simulink model "Galvo_sys_cc_neu_norefs_v32"  (R2013a)
settings: Solver=ode23  StartTime=0.0  StopTime=5e-3  MaxStep=1e-5  RelTol=1e-4  AbsTol=1e-6
PreLoadFcn:
  | paramCtrl=evalin('base','paramCtrl;');
  | 
  | I_LIM=str2num(paramCtrl.I_LIM);
  | Kbc=str2num(paramCtrl.Kbc);
InitFcn:
  | %I_LIM=str2num(paramCtrl.I_LIM);
  | %Kbc=str2num(paramCtrl.Kbc);
StartFcn:
  | %I_LIM=str2num(paramCtrl.I_LIM);
  | %Kbc=str2num(paramCtrl.Kbc);
values from neighbouring files (symbols this model uses):
  Lc = 170e-6    (= 0.00017)    [Galvo_process_analyze.m]
  Rc = 1.5    [Galvo_process_analyze.m]
undefined symbols (not defined in the file or in its folder): JR, KBM, KFR, KMT, KTB, Rsh
libraries: simulink x3
settings Model: BufferReuse=off  Creator=mainster  LastModifiedBy=mainster
settings SolverCC: MaxConsecutiveMinStep=2
settings OptimizationCC: BlockReduction=off  OptimizeBlockIOStorage=off  BufferReuse=off  ExpressionFolding=off  LocalBlockOutputs=off
settings ModelReferenceCC: ModelReferenceNumInstancesAllowed=Single

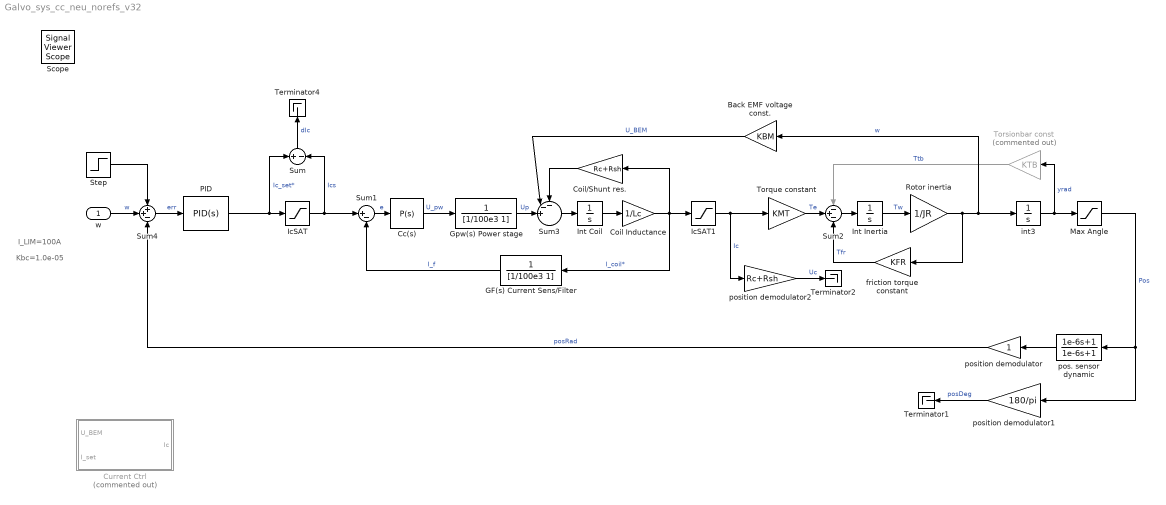
== system Galvo_sys_cc_neu_norefs_v32 ==
  note: I_LIM=100A
  note: Kbc=1.0e-05
  w : Inport
  Back EMF voltage const. : Gain  Gain=KBM
  Cc(s) : simulink/Continuous/PID Controller  Controller=P  TimeDomain=Continuous-time  SampleTime=1  IntegratorMethod=Forward Euler  FilterMethod=Forward Euler  Form=Ideal  P=5.91984122843419  I=14540.01765706  D=0  N=100  InitialConditionSource=internal  InitialConditionForIntegrator=0  InitialConditionForFilter=0  ExternalReset=none  LimitOutput=off  UpperSaturationLimit=inf  LowerSaturationLimit=-inf  LinearizeAsGain=on  AntiWindupMode=none  Kb=1  TrackingMode=off  Kt=1  PParamMin=[]  PParamMax=[]  IParamMin=[]  IParamMax=[]  DParamMin=[]  DParamMax=[]  NParamMin=[]  NParamMax=[]  KbParamMin=[]  KbParamMax=[]  KtParamMin=[]  KtParamMax=[]  POutMin=[]  POutMax=[]  IOutMin=[]  IOutMax=[]  DOutMin=[]  DOutMax=[]  NOutMin=[]  NOutMax=[]  KbOutMin=[]  KbOutMax=[]  KtOutMin=[]  KtOutMax=[]  IntegratorOutMin=[]  IntegratorOutMax=[]  FilterOutMin=[]  FilterOutMax=[]  SumOutMin=[]  SumOutMax=[]  SumI1OutMin=[]  SumI1OutMax=[]  SumI2OutMin=[]  SumI2OutMax=[]  SumI3OutMin=[]  SumI3OutMax=[]  SumDOutMin=[]  SumDOutMax=[]  SaturationOutMin=[]  SaturationOutMax=[]  IntegratorContinuousStateAttributes=''  IntegratorStateMustResolveToSignalObject=off  IntegratorRTWStateStorageClass=Auto  FilterContinuousStateAttributes=''  FilterStateMustResolveToSignalObject=off  FilterRTWStateStorageClass=Auto
  Coil Inductance : Gain  Gain=1/Lc
  Coil/Shunt res. : Gain  Gain=Rc+Rsh
  Current Ctrl : Subsystem  Commented=on
  GF(s) Current Sens/Filter : TransferFcn  Denominator=[1/100e3 1]
  Gpw(s) Power stage : TransferFcn  Denominator=[1/100e3 1]
  IcSAT : Saturate  UpperLimit=I_LIM  LowerLimit=-I_LIM
  IcSAT1 : Saturate  UpperLimit=I_LIM  LowerLimit=-I_LIM
  Int Coil : Integrator
  Int Inertia : Integrator
  Max Angle : Saturate  UpperLimit=20*pi/180  LowerLimit=-20*pi/180
      settings: AttributesFormatString=Max=%<UpperLimit>\nMin=%<LowerLimit>
  PID : simulink/Continuous/PID Controller  Controller=PID  TimeDomain=Continuous-time  SampleTime=1  IntegratorMethod=Forward Euler  FilterMethod=Forward Euler  Form=Ideal  P=5.80637204199794  I=20.9623797027831  D=0.0037150147392085  N=9551.68244277248  InitialConditionSource=internal  InitialConditionForIntegrator=0  InitialConditionForFilter=0  ExternalReset=none  IgnoreLimit=on  LimitOutput=off  UpperSaturationLimit=I_LIM*1e3  LowerSaturationLimit=-I_LIM*1e3  LinearizeAsGain=off  AntiWindupMode=back-calculation  Kb=Kbc  TrackingMode=off  Kt=0  PParamMin=[]  PParamMax=[]  IParamMin=[]  IParamMax=[]  DParamMin=[]  DParamMax=[]  NParamMin=[]  NParamMax=[]  KbParamMin=[]  KbParamMax=[]  KtParamMin=[]  KtParamMax=[]  POutMin=[]  POutMax=[]  IOutMin=[]  IOutMax=[]  DOutMin=[]  DOutMax=[]  NOutMin=[]  NOutMax=[]  KbOutMin=[]  KbOutMax=[]  KtOutMin=[]  KtOutMax=[]  IntegratorOutMin=[]  IntegratorOutMax=[]  FilterOutMin=[]  FilterOutMax=[]  SumOutMin=[]  SumOutMax=[]  SumI1OutMin=[]  SumI1OutMax=[]  SumI2OutMin=[]  SumI2OutMax=[]  SumI3OutMin=[]  SumI3OutMax=[]  SumDOutMin=[]  SumDOutMax=[]  SaturationOutMin=[]  SaturationOutMax=[]  IntegratorContinuousStateAttributes=''  IntegratorStateMustResolveToSignalObject=off  IntegratorRTWStateStorageClass=Auto  FilterContinuousStateAttributes=''  FilterStateMustResolveToSignalObject=off  FilterRTWStateStorageClass=Auto
      settings: AttributesFormatString=AWM=%<AntiWindupMode>\nD=%<D>\nI=%<I>\nN=%<N>\nP=%<P>\nLimit=+-%<UpperSaturationLimit>
  Rotor inertia : Gain  Gain=1/JR
  Step : Step  Time=1e-3  After=1*pi/180  SampleTime=0  ZeroCross=off
      settings: AttributesFormatString=Ampl.: %<After>
  Sum : Sum  Inputs=+-
  Sum1 : Sum  Inputs=|+-
  Sum2 : Sum  Inputs=-+-
  Sum3 : Sum  Inputs=--+||
  Sum4 : Sum  Inputs=++-
  Terminator1 : Terminator
  Terminator2 : Terminator
  Terminator4 : Terminator
  Torque constant : Gain  Gain=KMT
  Torsionbar const : Gain  Commented=on  Gain=KTB
  friction torque constant : Gain  Gain=KFR
  int3 : Integrator
  pos. sensor dynamic : TransferFcn  Numerator=[1e-6 1]  Denominator=[1e-6 1]
  position demodulator : Gain
  position demodulator1 : Gain  Gain=180/pi
  position demodulator2 : Gain  Gain=Rc+Rsh
  Scope : SignalViewerScope  IOType=viewer  NumInputPorts=5  RefreshTime=0.035000
      settings: ShowLegends=on  TimeRange=0.005  YMin=-10~-10~-1~0~-5  YMax=40~50~1~0.2~15
  wires:
  Sum4/1 -> PID/1  "err"
  Step/1 -> Sum4/1
  w/1 -> Sum4/2  "w"
  pos. sensor dynamic/1 -> position demodulator/1
  position demodulator/1 -> Sum4/3  "posRad"
  Max Angle/1 -> position demodulator1/1, pos. sensor dynamic/1  "Pos"
  PID/1 -> Sum/1, IcSAT/1  "Ic_set*"
  Coil Inductance/1 -> IcSAT1/1, Coil/Shunt res./1, GF(s) Current Sens/Filter/1  "I_coil*"
  position demodulator1/1 -> Terminator1/1  "posDeg"
  position demodulator2/1 -> Terminator2/1  "Uc"
  Sum/1 -> Terminator4/1  "dIc"
  IcSAT/1 -> Sum1/1, Sum/2  "Ics"
  Sum1/1 -> Cc(s)/1  "e"
  Coil/Shunt res./1 -> Sum3/1
  Sum3/1 -> Int Coil/1
  Int Coil/1 -> Coil Inductance/1
  Cc(s)/1 -> Gpw(s) Power stage/1  "U_pw"
  Gpw(s) Power stage/1 -> Sum3/3  "Up"
  GF(s) Current Sens/Filter/1 -> Sum1/2  "I_f"
  int3/1 -> Max Angle/1, Torsionbar const/1  "yrad"
  Torque constant/1 -> Sum2/2  "Te"
  Torsionbar const/1 -> Sum2/1  "Ttb"
  Int Inertia/1 -> Rotor inertia/1  "Tw"
  Sum2/1 -> Int Inertia/1
  Rotor inertia/1 -> int3/1, Back EMF voltage const./1, friction torque constant/1  "w"
  friction torque constant/1 -> Sum2/3  "Tfr"
  IcSAT1/1 -> Torque constant/1, position demodulator2/1  "Ic"
  Back EMF voltage const./1 -> Sum3/2  "U_BEM"

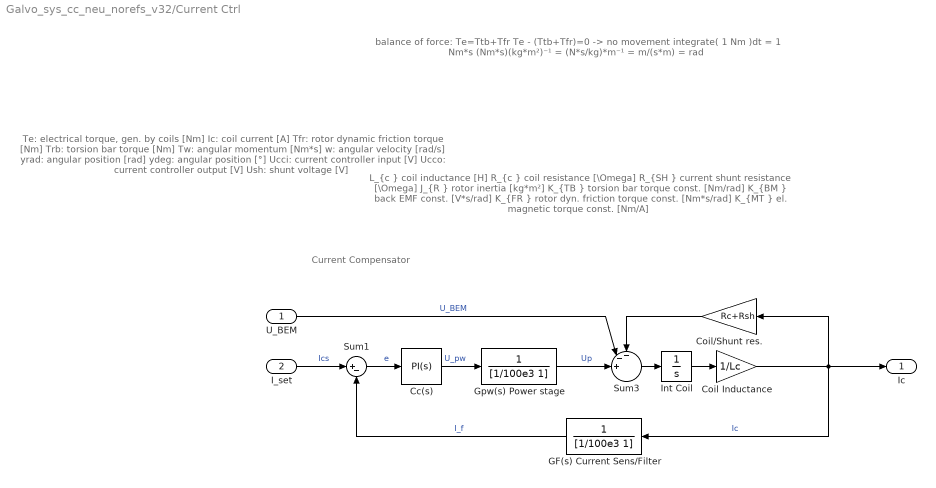
== system Galvo_sys_cc_neu_norefs_v32/Current Ctrl ==
  note: Current Compensator
  note: Te: 		electrical torque, gen. by coils		[Nm]
      |  Ic: 			coil current							[A]
      |  Tfr:		rotor dynamic friction torque 		[Nm]
      |  Trb:		torsion bar torque					[Nm]
      |  Tw:		angular momentum				[Nm*s]
      |  w:			angular velocity 					[rad/s]
      |  yrad:		angular position 					[rad]
      |  ydeg:		angular position 					[°]
      |  Ucci:		current controller input				[V]
      |  Ucco:		current controller output			[V]
      |  Ush:		shunt voltage						[V]
  note: L_{c  }	coil inductance 							[H]
      |  R_{c  }	coil resistance							[\Omega]
      |  R_{SH }	current shunt resistance				[\Omega]
      |  J_{R  }	rotor inertia 							[kg*m²]
      |  K_{TB }	torsion bar torque const. 			[Nm/rad]
      |  K_{BM }	back EMF const.							[V*s/rad]
      |  K_{FR }	rotor dyn. friction torque const.	[Nm*s/rad]
      |  K_{MT }	el. magnetic torque const.			[Nm/A]
  note: balance of force: 	Te=Ttb+Tfr
      | 					Te - (Ttb+Tfr)=0  ->  no movement
      |
      |  integrate( 1 Nm )dt = 1 Nm*s
      |  (Nm*s)(kg*m²)⁻¹ = (N*s/kg)*m⁻¹ = m/(s*m) = rad
  U_BEM : Inport
  I_set : Inport  Port=2
  Cc(s) : simulink/Continuous/PID Controller  Controller=PI  TimeDomain=Continuous-time  SampleTime=1  IntegratorMethod=Forward Euler  FilterMethod=Forward Euler  Form=Ideal  P=2.58986900309333  I=14540.01765706  D=0  N=100  InitialConditionSource=internal  InitialConditionForIntegrator=0  InitialConditionForFilter=0  ExternalReset=none  LimitOutput=off  UpperSaturationLimit=inf  LowerSaturationLimit=-inf  LinearizeAsGain=on  AntiWindupMode=none  Kb=1  TrackingMode=off  Kt=1  PParamMin=[]  PParamMax=[]  IParamMin=[]  IParamMax=[]  DParamMin=[]  DParamMax=[]  NParamMin=[]  NParamMax=[]  KbParamMin=[]  KbParamMax=[]  KtParamMin=[]  KtParamMax=[]  POutMin=[]  POutMax=[]  IOutMin=[]  IOutMax=[]  DOutMin=[]  DOutMax=[]  NOutMin=[]  NOutMax=[]  KbOutMin=[]  KbOutMax=[]  KtOutMin=[]  KtOutMax=[]  IntegratorOutMin=[]  IntegratorOutMax=[]  FilterOutMin=[]  FilterOutMax=[]  SumOutMin=[]  SumOutMax=[]  SumI1OutMin=[]  SumI1OutMax=[]  SumI2OutMin=[]  SumI2OutMax=[]  SumI3OutMin=[]  SumI3OutMax=[]  SumDOutMin=[]  SumDOutMax=[]  SaturationOutMin=[]  SaturationOutMax=[]  IntegratorContinuousStateAttributes=''  IntegratorStateMustResolveToSignalObject=off  IntegratorRTWStateStorageClass=Auto  FilterContinuousStateAttributes=''  FilterStateMustResolveToSignalObject=off  FilterRTWStateStorageClass=Auto
  Coil Inductance : Gain  Gain=1/Lc
  Coil/Shunt res. : Gain  Gain=Rc+Rsh
  GF(s) Current Sens/Filter : TransferFcn  Denominator=[1/100e3 1]
  Gpw(s) Power stage : TransferFcn  Denominator=[1/100e3 1]
  Int Coil : Integrator
  Sum1 : Sum  Inputs=|+-
  Sum3 : Sum  Inputs=--+||
  Ic : Outport
  wires:
  Cc(s)/1 -> Gpw(s) Power stage/1  "U_pw"
  GF(s) Current Sens/Filter/1 -> Sum1/2  "I_f"
  Coil/Shunt res./1 -> Sum3/1
  Sum3/1 -> Int Coil/1
  Gpw(s) Power stage/1 -> Sum3/3  "Up"
  Coil Inductance/1 -> Ic/1, GF(s) Current Sens/Filter/1, Coil/Shunt res./1  "Ic"
  I_set/1 -> Sum1/1  "Ics"
  Sum1/1 -> Cc(s)/1  "e"
  Int Coil/1 -> Coil Inductance/1
  U_BEM/1 -> Sum3/2  "U_BEM"
